simulink model "mean_and_std_dev"  (R2022b)
settings: Solver=VariableStepAuto  StartTime=0.0  StopTime=10.0  RelTol=1e-3
settings Model: Creator=Brigosha_Guest  LastModifiedBy=Brigosha_Guest

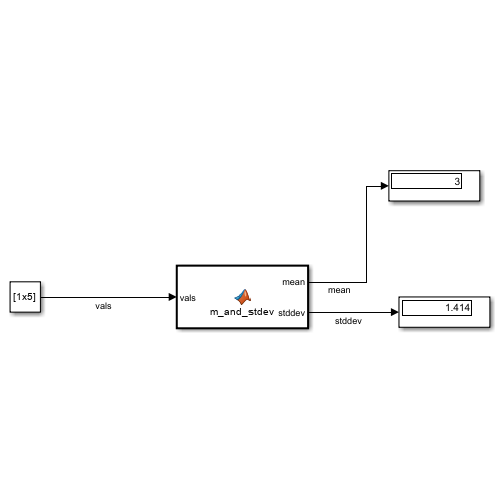
[thumbnail: Simulink's stored preview of the top-level diagram]
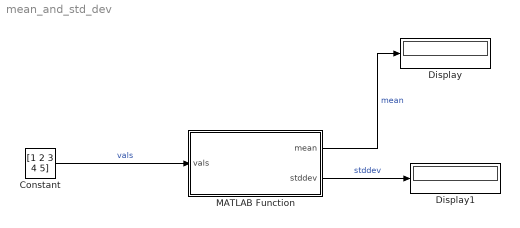
== system mean_and_std_dev ==
  Constant : Constant  Value=[1 2 3 4 5]
  Display : Display
  Display1 : Display
  MATLAB Function : MATLAB Function  TreatAsAtomicUnit=on
  wires:
  Constant/1 -> MATLAB Function/1(vals)  "vals"
  MATLAB Function/1(mean) -> Display/1  "mean"
  MATLAB Function/2(stddev) -> Display1/1  "stddev"

== matlab function mean_and_std_dev/MATLAB Function ==
  data: vals input; mean output; stddev output
function [mean, stddev] = m_and_stdev(vals)
len=length(vals);
s=sum(vals);
mean=s/len;
stddev=sqrt(sum((vals-mean).^2)/len);
end
